simulink model "resp"  (R2016a)
settings: Solver=VariableStepAuto  StartTime=0.0  StopTime=10.0  RelTol=1e-3
values from neighbouring files (symbols this model uses):
  dt = 0.005    [main.m]
  MC = MI*CC    [main.m]
  MF = inv(M)*F    [main.m]
settings Model: Creator=Geraldo  LastModifiedBy=Geraldo
settings DataIOCC: SaveFormat=Array

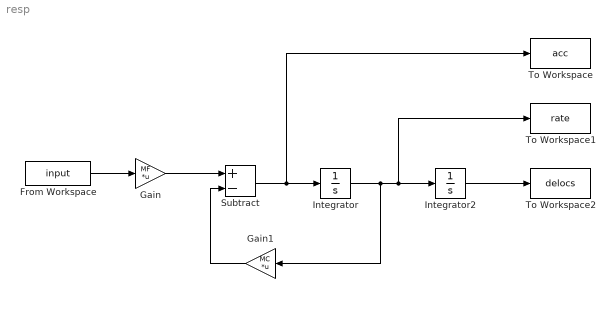
== system resp ==
  From Workspace : FromWorkspace  VariableName=input  SampleTime=dt
  Gain : Gain  Gain=MF  Multiplication=Matrix(K*u)
  Gain1 : Gain  Gain=MC  Multiplication=Matrix(K*u)
  Integrator : Integrator
  Integrator2 : Integrator
  Subtract : Sum  Inputs=+-
  To Workspace : ToWorkspace  VariableName=acc  SampleTime=dt
  To Workspace1 : ToWorkspace  VariableName=rate  SampleTime=dt
  To Workspace2 : ToWorkspace  VariableName=delocs  SampleTime=dt
  wires:
  From Workspace/1 -> Gain/1
  Gain/1 -> Subtract/1
  Gain1/1 -> Subtract/2
  Integrator2/1 -> To Workspace2/1
  Subtract/1 -> Integrator/1, To Workspace/1
  Integrator/1 -> Gain1/1, To Workspace1/1, Integrator2/1
